simulink model "VG_Main"  (R2024b)
settings: Solver=VariableStepAuto  StartTime=0.0  StopTime=1  FixedStep=1e-3  MaxStep=1e-4  RelTol=1e-3
libraries: cstblocks x1
settings Model: SimulationMode=accelerator  Creator=luigi  LastModifiedBy=luigi

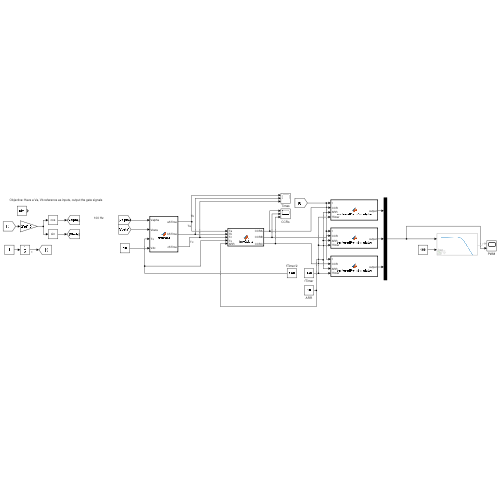
[thumbnail: Simulink's stored preview of the top-level diagram]
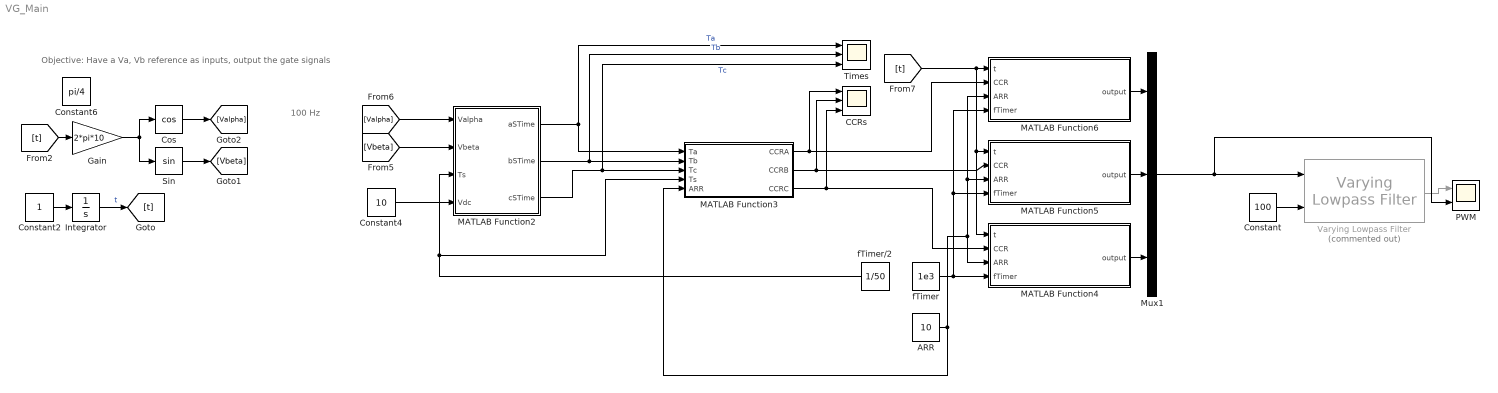
== system VG_Main ==
  note: 100 Hz
  note: Objective: Have a Va, Vb reference as inputs, output the gate signals
  ARR : Constant  Value=10
  CCRs : Scope  NumInputPorts=3
  Constant : Constant  Value=100
  Constant2 : Constant
  Constant4 : Constant  Value=10
  Constant6 : Constant  Value=pi/4
  Cos : Trigonometry  Operator=cos
  Gain : Gain  Gain=2*pi*10
  Integrator : Integrator
  MATLAB Function2 : MATLAB Function  TreatAsAtomicUnit=on
  MATLAB Function3 : MATLAB Function  TreatAsAtomicUnit=on
  MATLAB Function4 : MATLAB Function  TreatAsAtomicUnit=on
  MATLAB Function5 : MATLAB Function  TreatAsAtomicUnit=on
  MATLAB Function6 : MATLAB Function  TreatAsAtomicUnit=on
  Mux1 : Mux  Inputs=3
  PWM : Scope  NumInputPorts=2
  Sin : Trigonometry
  Times : Scope  NumInputPorts=3
  Varying Lowpass Filter : cstblocks/Linear Parameter Varying/Varying Lowpass Filter  Commented=on  N=1
  fTimer : Constant  Value=1e3
  fTimer/2 : Constant  Value=1/50
  wires:
  fTimer/2/1 -> MATLAB Function2/3(Ts), MATLAB Function3/4(Ts)
  Constant2/1 -> Integrator/1
  Constant/1 -> Varying Lowpass Filter/2
  Integrator/1 -> [t]  "t"
  [t] -> Gain/1
  Sin/1 -> [Vbeta]
  Cos/1 -> [Valpha]
  Constant4/1 -> MATLAB Function2/4(Vdc)
  [Vbeta] -> MATLAB Function2/2(Vbeta)
  [Valpha] -> MATLAB Function2/1(Valpha)
  MATLAB Function2/2(bSTime) -> Times/2, MATLAB Function3/2(Tb)  "Tb"
  MATLAB Function2/3(cSTime) -> Times/3, MATLAB Function3/3(Tc)  "Tc"
  MATLAB Function2/1(aSTime) -> MATLAB Function3/1(Ta), Times/1  "Ta"
  [t] -> MATLAB Function5/1(t), MATLAB Function4/1(t), MATLAB Function6/1(t)
  MATLAB Function3/1(CCRA) -> CCRs/1, MATLAB Function6/2(CCR)
  ARR/1 -> MATLAB Function4/3(ARR), MATLAB Function5/3(ARR), MATLAB Function6/3(ARR), MATLAB Function3/5(ARR)
  MATLAB Function3/2(CCRB) -> MATLAB Function5/2(CCR), CCRs/2
  MATLAB Function3/3(CCRC) -> MATLAB Function4/2(CCR), CCRs/3
  fTimer/1 -> MATLAB Function4/4(fTimer), MATLAB Function5/4(fTimer), MATLAB Function6/4(fTimer)
  Gain/1 -> Cos/1, Sin/1
  Varying Lowpass Filter/1 -> PWM/1
  MATLAB Function5/1(output) -> Mux1/2
  MATLAB Function6/1(output) -> Mux1/1
  MATLAB Function4/1(output) -> Mux1/3
  Mux1/1 -> PWM/2, Varying Lowpass Filter/1

== matlab function VG_Main/MATLAB Function2 ==
  data: Valpha input; aSTime output; Vbeta input; Ts input; Vdc input; bSTime output; cSTime output
function [aSTime, bSTime, cSTime] = SVPWM(Valpha, Vbeta, Ts, Vdc)

piThird = pi/3;
scaling = 2/sqrt(3);


% First step: determine the angle of the reference
theta = atan(Vbeta/Valpha);

if(theta < 0)
    theta = theta + pi;
end

if(Vbeta < 0)
    theta = theta + pi;
end

Vref = sqrt(Valpha*Valpha+Vbeta*Vbeta);

quad = ceil(theta/piThird);

modulation = (3/2) * (Vref/Vdc);

ThB = (quad-1) * piThird; %Angle of first possible vector
ThA = quad * piThird; %Angle of the second vector

Ta = scaling * modulation * Ts * sin(ThA - theta);
Tb = scaling * modulation * Ts * sin(theta - ThB);
Tz = Ts - Ta - Tb;

aSTime = 0;
bSTime = 0;
cSTime = 0;

switch quad
    case 1
        aSTime = Ta + Tb + Tz/2;
        bSTime = Tb + Tz/2;
        cSTime = Tz/2;
    case 2
        aSTime = Ta + Tz/2;
        bSTime  = Ta + Tb + Tz/2;
        cSTime  = Tz/2;
    case 3
        aSTime = Tz/2;
        bSTime = Ta + Tb + Tz/2;
        cSTime  = Tb + Tz/2;
    case 4
        aSTime = Tz/2;
        bSTime = Ta + Tz/2;
        cSTime  = Ta + Tb + Tz/2;
    case 5
        aSTime = Tb + Tz/2;
        bSTime = Tz/2;
        cSTime = Ta + Tb + Tz/2;
    case 6
        aSTime  = Ta + Tb + Tz/2;
        bSTime = Tz/2;
        cSTime = Ta + Tz/2;
end

== matlab function VG_Main/MATLAB Function3 ==
  data: Ta input; Tb input; Tc input; CCRA output; Ts input; CCRB output; CCRC output; ARR input
function [CCRA, CCRB, CCRC] = time2duty(Ta, Tb, Tc, Ts, ARR)
% This function converts switching times to CCR values for timers
% set in PWM Mode 3 - Center Aligned

dcA = Ta / Ts;
dcB = Tb / Ts;
dcC = Tc / Ts;

% CCRA / ARR = dcA;
CCRA = ARR * (1-dcA);
CCRB = ARR * (1-dcB);
CCRC = ARR * (1-dcC);
end

== matlab function VG_Main/MATLAB Function4 ==
  settings: updateMethod=DISCRETE
  data: t input; output output; CCR input; ARR input; fTimer input
function output  = centeredPwmSimulator(t, CCR, ARR, fTimer)
% This function aims to emulate the behaviour of a single channel
% of the STM32 PWM hardware 

Ts = 1/fTimer;

persistent counter
persistent timeCounter
persistent direction
persistent outState
if isempty(outState)
    outState = 0;
end
if isempty(timeCounter)
    timeCounter = 0;
end
if isempty(counter)
    counter = 0;
end
if isempty(direction)
    direction = 1;
end

if (t - timeCounter * Ts) > 0
    delta = 1;
    timeCounter = timeCounter + 1;
else 
    delta = 0;
end

if counter >= ARR
    direction = -1;
end
if counter <= 0
    direction = 1;
end

counter = counter + delta .* direction;

if(counter == round(CCR) && delta ~= 0)
    if(outState == 0)
        outState = 1;
    else
        outState = 0;
    end
end

output = outState;

end

== matlab function VG_Main/MATLAB Function5 ==
  settings: updateMethod=DISCRETE
  data: t input; output output; CCR input; ARR input; fTimer input
function output  = centeredPwmSimulator(t, CCR, ARR, fTimer)
% This function aims to emulate the behaviour of a single channel
% of the STM32 PWM hardware 

Ts = 1/fTimer;

persistent counter
persistent timeCounter
persistent direction
persistent outState
if isempty(outState)
    outState = 0;
end
if isempty(timeCounter)
    timeCounter = 0;
end
if isempty(counter)
    counter = 0;
end
if isempty(direction)
    direction = 1;
end

if (t - timeCounter * Ts) > 0
    delta = 1;
    timeCounter = timeCounter + 1;
else 
    delta = 0;
end

if counter >= ARR
    direction = -1;
end
if counter <= 0
    direction = 1;
end

counter = counter + delta .* direction;

if(counter == round(CCR) && delta ~= 0)
    if(outState == 0)
        outState = 1;
    else
        outState = 0;
    end
end

output = outState;

end

== matlab function VG_Main/MATLAB Function6 ==
  settings: updateMethod=DISCRETE
  data: t input; output output; CCR input; ARR input; fTimer input
function output  = centeredPwmSimulator(t, CCR, ARR, fTimer)
% This function aims to emulate the behaviour of a single channel
% of the STM32 PWM hardware 

Ts = 1/fTimer;

persistent counter
persistent timeCounter
persistent direction
persistent outState
if isempty(outState)
    outState = 0;
end
if isempty(timeCounter)
    timeCounter = 0;
end
if isempty(counter)
    counter = 0;
end
if isempty(direction)
    direction = 1;
end

if (t - timeCounter * Ts) > 0
    delta = 1;
    timeCounter = timeCounter + 1;
else 
    delta = 0;
end

if counter >= ARR
    direction = -1;
end
if counter <= 0
    direction = 1;
end

counter = counter + delta .* direction;

if(counter == round(CCR) && delta ~= 0)
    if(outState == 0)
        outState = 1;
    else
        outState = 0;
    end
end

output = outState;

end
